simulink model "Coffe_vending_Machine"  (R2020b)
settings: Solver=FixedStepDiscrete  StartTime=0.0  StopTime=200  RelTol=1e-3
settings Model: Creator=The MathWorks, Inc.  LastModifiedBy=intel
settings DataIOCC: LimitDataPoints=on  SaveFormat=Array  ReturnWorkspaceOutputs=off
settings OptimizationCC: ExpressionDepthLimit=2147483647  InitFltsAndDblsToZero=on  EfficientMapNaN2IntZero=off  LifeSpan=inf
settings DebuggingCC: SaveWithParameterizedLinksMsg=none  UnderspecifiedInitializationDetection=Classic  MergeDetectMultiDrivingBlocksExec=none  SignalResolutionControl=TryResolveAllWithWarning  SolverPrmCheckMsg=warning  MultiTaskDSMMsg=warning  MultiTaskCondExecSysMsg=none  FcnCallInpInsideContextMsg=warning  StateNameClashWarn=warning  SFUnexpectedBacktrackingDiag=warning  SFNoUnconditionalDefaultTransitionDiag=warning  SFExecutionAtInitializationDiag=none  ArithmeticOperatorsInVariantConditions=warning
settings HardwareCC: ProdBitPerPointer=32  ProdBitPerSizeT=32  ProdBitPerPtrDiffT=32  ProdLargestAtomicFloat=None  ProdIntDivRoundTo=Undefined  ProdEndianess=Unspecified  ProdWordSize=32  ProdHWDeviceType=32-bit Generic
settings ModelReferenceCC: PropagateSignalLabelsOutOfModel=off
settings SFSimCC: SimUseLocalCustomCode=off  SimParseCustomCode=off  CustomCodeUndefinedFunction=UseInterfaceOnly
settings RTWCC: RTWUseLocalCustomCode=off
settings CodeAppCC: StateflowObjectComments=on
settings GRTTargetCC: TargetFcnLib=ansi_tfl_tmw.mat  TargetLangStandard=C89/C90 (ANSI)  CombineOutputUpdateFcns=off  GRTInterface=on
settings ConfigComp: CovMetricSettings=dw  CovSaveCumulativeToWorkspaceVar=on  CovSaveSingleToWorkspaceVar=on  CovExternalEMLEnable=off  CovSFcnEnable=off

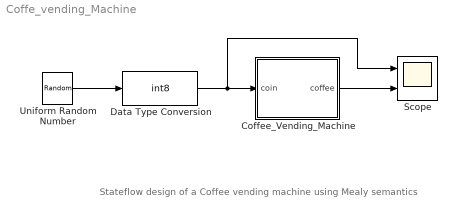
== system Coffe_vending_Machine ==
  note: Stateflow design of a Coffee vending machine using Mealy semantics
  " Data Type Conversion" : DataTypeConversion  OutDataTypeStr=int8  RndMeth=Nearest  SaturateOnIntegerOverflow=on
  " Scope" : Scope  NumInputPorts=2
  " Uniform Random Number" : UniformRandomNumber  Minimum=0  Maximum=2  Seed=337  SampleTime=10
  Coffee_Vending_Machine : Stateflow chart  TreatAsAtomicUnit=on
  wires:
  " Uniform Random Number"/1 -> " Data Type Conversion"/1
  " Data Type Conversion"/1 -> Coffee_Vending_Machine/1(coin), " Scope"/1
  Coffee_Vending_Machine/1(coffee) -> " Scope"/2

== stateflow chart Coffe_vending_Machine/Coffee_Vending_Machine ==
  settings: stateMachineType=MEALY_MACHINE  initializeOutput=1
  state got_coffee
  state got_milk_sugar
  state got_coffee_powder
  (default) -> got_coffee
  got_coffee -> got_milk_sugar [order 1] : [coin==1]{coffee=0}
  got_milk_sugar -> got_coffee [order 2] : [coin==2]{coffee=1}
  got_coffee_powder -> got_coffee [order 1] : [coin==1]{coffee=1}
  got_coffee -> got_coffee_powder [order 2] : [coin==2]{coffee=0}
  got_milk_sugar -> got_coffee_powder [order 1] : [coin==1]{coffee=0}
  got_coffee_powder -> got_milk_sugar [order 2] : [coin==2]{coffee=1}
  data: coin input int8; coffee output double
